simulink model "Consigna5_2_1"  (R2024b)
settings: Solver=ode45  StartTime=0.0  StopTime=20  RelTol=1e-3
values from neighbouring files (symbols this model uses):
  A_corrientes = [0 1; -omega_n_corrientes^2 -2*omega_n_corrientes]    [parametros.m]
  A_inversor = [0 1; -omega_n_inversor^2 -2*omega_n_inversor]    [parametros.m]
  A_posicion = [0 1; -omega_n_posicion^2 -2*omega_n_posicion]    [parametros.m]
  A_temp = -1/20    (= -0.05)    [parametros.m]
  alpha_cu = 3.9 *10^-3    (= 0.0039)    [parametros.m]
  B_corrientes = [0; omega_n_corrientes^2]    [parametros.m]
  b_eq = b_m + (1/r^2) * b_l    (= 2.19444444444e-05)    [parametros.m]
  B_inversor = [0; omega_n_inversor^2]    [parametros.m]
  b_l = 0.1    [parametros.m]
  b_m = 1.5 * 10^-5    (= 1.5e-05)    [parametros.m]
  B_posicion = [0; omega_n_posicion^2]    [parametros.m]
  B_temp = 1/20    (= 0.05)    [parametros.m]
  ba = J_eq*n*omega_pos    (= 0.0916527777778)    [parametros.m]
  C_corrientes = [1 0]    [parametros.m]
  C_inversor = [1 0]    [parametros.m]
  C_posicion = [1 0]    [parametros.m]
  C_temp = 1    [parametros.m]
  C_ts = 0.818    [parametros.m]
  g = 9.80665    [parametros.m]
  J_l = (m*l_cm^2 + J_cm) + (m_l * l_l^2)    (= 0.4583)    [parametros.m]
  J_m = 1.4 * 10^-5    (= 1.4e-05)    [parametros.m]
  K_e_int = 3200 ^3    (= 32768000000)    [parametros.m]
  K_e_omega = 3*3200^2    (= 30720000)    [parametros.m]
  K_e_theta = 9600    [parametros.m]
  k_l = m * l_cm + m_l* l_l    (= 1)    [parametros.m]
  Ksa = J_eq*n*(omega_pos^2)    (= 73.3222222222)    [parametros.m]
  Ksia = J_eq*(omega_pos^3)    (= 23463.1111111)    [parametros.m]
  L_d = 6.6 * 10^-3    (= 0.0066)    [parametros.m]
  L_ls = 0.8 * 10^-3    (= 0.0008)    [parametros.m]
  L_q = 5.8 * 10^-3    (= 0.0058)    [parametros.m]
  lambda_m = 0.016    [parametros.m]
  P_p = 3    [parametros.m]
  r = 120    [parametros.m]
  R_s_40 = 1.02    [parametros.m]
  R_ts_amb = 146.7    [parametros.m]
  T_sample = 1/f_sample    (= 4.53514739229e-05)    [parametros.m]
  Temp_s_ref = 20    [parametros.m]
  tm = X(1)    [parametros.m]
  tr = X(2)    [parametros.m]
  w2 = 188.49556    [parametros.m]
  x0_corrientes = [0;0]    [parametros.m]
  x0_inversor = [0;0]    [parametros.m]
  x0_posicion = [0; 0]    [parametros.m]
  x0_temp = 20    [parametros.m]
libraries: simulink x14, dspsigops x6
(part 1 of 4)
settings Model: Creator=nsorr  LastModifiedBy=nsorr
settings SolverCC: ZeroCrossAlgorithm=Adaptive
settings DebuggingCC: IgnoredZcDiagnostic=none

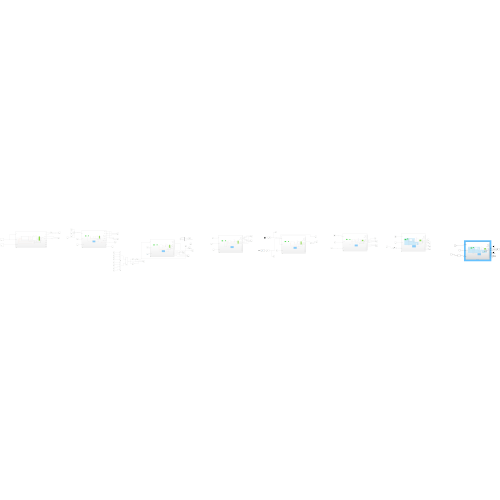
[thumbnail: Simulink's stored preview of the top-level diagram]
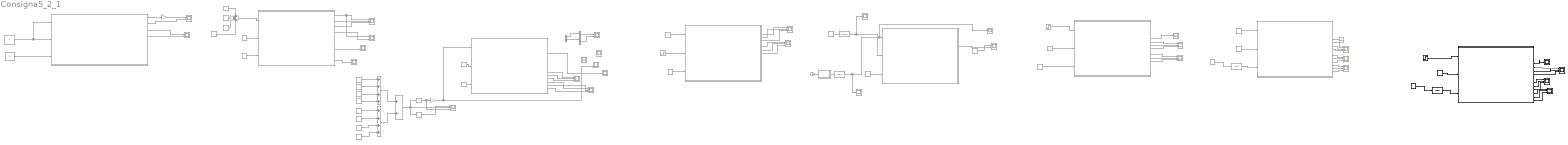
== system Consigna5_2_1 ==
  .5s : Step  Time=.5  After=5  SampleTime=0
  0-5 : simulink/Sources/Ramp  Commented=on  slope=2*pi/5  start=0  InitialOutput=0
  10-15 : simulink/Sources/Ramp  Commented=on  slope=-2*pi/5  start=10  InitialOutput=0
  5-10 : simulink/Sources/Ramp  Commented=on  slope=-2*pi/5  start=5  InitialOutput=0
  Clock : Clock  Commented=on
  Constant{,3,5..6,10,16} (6 alike) : Constant  Commented=on  Value=0
  Constant{1..2,4,7,9,11,13} (7 alike) : Constant  Commented=on  Value=20
  Constant14 : Constant  Value=20
  Constant8 : Constant  Commented=on  Value=115
  Demux2 : Demux  Commented=on  Outputs=2
  Derivative1 : Derivative  Commented=on
  Error de observador2 : Scope  Commented=on  NumInputPorts=2
  Gain : Gain  Commented=on  Gain=1/r
  Gain1 : Gain  Commented=on  Gain=1/r
  Integrator1 : Integrator  Commented=on
  MATLAB Function : MATLAB Function  Commented=on  TreatAsAtomicUnit=on
  Mux10 : Mux  Commented=on  Inputs=2
  Mux8 : Mux  Commented=on  Inputs=2
  Pulse Generator : DiscretePulseGenerator  Commented=on  PulseType=Time based  Amplitude=5  Period=1  PulseWidth=50
  Ramp : simulink/Sources/Ramp  Commented=on  slope=2*pi/5  start=15  InitialOutput=0
  Ramp1 : simulink/Sources/Ramp  Commented=on  slope=3*pi  start=5  InitialOutput=0
  Ramp10 : simulink/Sources/Ramp  Commented=on  slope=w2  start=10+tr+tm  InitialOutput=0
  Ramp11 : simulink/Sources/Ramp  Commented=on  slope=w2  start=10+tr  InitialOutput=0
  Ramp12 : simulink/Sources/Ramp  Commented=on  slope=w2  start=0  InitialOutput=0
  Ramp13 : simulink/Sources/Ramp  Commented=on  slope=-w2  start=10  InitialOutput=0
  Ramp14 : simulink/Sources/Ramp  Commented=on  slope=w2  start=5  InitialOutput=0
  Ramp15 : simulink/Sources/Ramp  Commented=on  slope=-w2  start=tr  InitialOutput=0
  Ramp16 : simulink/Sources/Ramp  Commented=on  slope=-w2  start=tr+tm  InitialOutput=0
  Ramp2 : simulink/Sources/Ramp  slope=3*pi  start=5  InitialOutput=0
  Ramp9 : simulink/Sources/Ramp  Commented=on  slope=-w2  start=15  InitialOutput=0
  Scope{,1,3..4,12} (5 alike) : Scope  Commented=on  NumInputPorts=2
  Scope{5,9..11,14,16} (6 alike) : Scope  Commented=on
  Scope{2,6..8,13,15} (6 alike) : Scope  Commented=on  NumInputPorts=3
  Scope17 : Scope  NumInputPorts=3
  Scope18 : Scope
  Step : Step  Commented=on  Time=7.5  After=5  SampleTime=0
  Step4 : Step  Commented=on  Time=7.5  After=5  SampleTime=0
  Subsystem : Subsystem  Commented=on
  Subsystem1 : Subsystem  Commented=on
  Subsystem2 : Subsystem  Commented=on
  Subsystem3 : Subsystem  Commented=on
  Subsystem4 : Subsystem  Commented=on
  Subsystem5 : Subsystem  Commented=on
  Subsystem6 : Subsystem  Commented=on
  Subsystem7 : Subsystem
  Sum : Sum  Commented=on  Inputs=++++
  Sum1 : Sum  Commented=on  Inputs=++++
  Sum2 : Sum  Commented=on  Inputs=++++
  Sum3 : Sum  Commented=on
  Transfer Fcn1 : TransferFcn  Numerator=[10]  Denominator=[1 10]
  Transfer Fcn3 : TransferFcn  Commented=on  Numerator=[100]  Denominator=[1 100]
  Transfer Fcn4 : TransferFcn  Commented=on  Numerator=[10]  Denominator=[1 10]
  Transfer Fcn8 : TransferFcn  Commented=on  Numerator=[20]  Denominator=[1 20]
  corrientes{1..4,6} (5 alike) : Scope  Commented=on  NumInputPorts=3
  corrientes5 : Scope  NumInputPorts=3
  corrientes7 : Scope  NumInputPorts=3
  posicion del brazo5 : Scope  Commented=on  NumInputPorts=2
  temp1 : Scope  Commented=on
  temp5 : Scope  Commented=on
  torque5 : Scope  Commented=on
  wires:
  Constant/1 -> Subsystem/2(T_per), Subsystem/1(Tm*)
  Constant1/1 -> Subsystem/3(T°_amb)
  Subsystem/1(T_l) -> Gain/1
  Gain/1 -> Scope/1  "T_l"
  Subsystem/2(T_m) -> Scope/2  "T_m"
  Subsystem/3(theta_m) -> Scope1/1  "theta_m"
  Subsystem/4(omega_m) -> Scope1/2  "omega_m"
  Constant2/1 -> Subsystem1/3(T°_amb)
  10-15/1 -> Sum/3
  Sum/1 -> Subsystem1/1(q1*)  "Consigna Articulación"
  Constant3/1 -> Subsystem1/2(T_per)
  0-5/1 -> Sum/1
  5-10/1 -> Sum/2
  Ramp/1 -> Sum/4
  Subsystem1/2(theta_m) -> Scope2/2  "theta_m"
  Subsystem1/7(T_m) -> Scope4/2  "Tm"
  Subsystem1/9(T_s) -> Scope5/1
  Subsystem1/4(omega_m*) -> Scope3/2  "omega_m*"
  Subsystem1/1(theta_m*) -> Scope3/1, Scope2/1  "theta_m*"
  Subsystem1/3(theta_m_obs) -> Scope2/3
  Constant4/1 -> Subsystem2/3(T°_amb)
  Constant5/1 -> Subsystem2/2(T_per)
  Ramp10/1 -> Sum1/2
  Ramp9/1 -> Sum1/1
  Ramp11/1 -> Sum1/3
  Ramp13/1 -> Sum1/4
  Ramp14/1 -> Sum2/1
  Ramp16/1 -> Sum2/2
  Ramp15/1 -> Sum2/3
  Ramp12/1 -> Sum2/4
  Sum2/1 -> Sum3/2
  Sum3/1 -> Scope8/2, Derivative1/1, Integrator1/1  "vel"
  Sum1/1 -> Sum3/1
  Integrator1/1 -> Scope8/3, Gain1/1  "Consigna de Posicion"
  Derivative1/1 -> Scope8/1  "acel"
  Mux10/1 -> Error de observador2/2
  Demux2/2 -> Mux10/1  "theta_m_obs"
  Mux8/1 -> Error de observador2/1
  Demux2/1 -> Mux8/1  "omega_m_obs"
  Subsystem2/4(T_s) -> temp5/1  "T_s"
  Gain1/1 -> posicion del brazo5/2, Subsystem2/1(q1*)
  Subsystem2/10(f_as) -> corrientes6/1  "i_as"
  Subsystem2/11(f_bs) -> corrientes6/2  "i_bs"
  Subsystem2/12(f_cs) -> corrientes6/3  "i_cs"
  Subsystem2/13(v_as) -> corrientes1/1
  Subsystem2/14(v_bs) -> corrientes1/2
  Subsystem2/15(v_cs) -> corrientes1/3
  Step4/1 -> Subsystem3/2(T_per)  "Tper"
  Constant6/1 -> Subsystem3/1(q1*)
  Constant7/1 -> Subsystem3/3(T°_amb)
  Subsystem3/8(theta_m_obs) -> Scope6/3  "theta_m_obs"
  Subsystem3/6(theta_m*) -> Scope6/1  "theta_m*"
  Subsystem3/7(theta_m) -> Scope6/2  "theta_m"
  Subsystem3/2(omega_m*) -> Scope7/1  "omega_m*"
  Subsystem3/3(omega_m) -> Scope7/2  "omega_m"
  Subsystem3/4(omega_m_obs) -> Scope7/3  "omega_m_obs"
  Clock/1 -> MATLAB Function/1(t)
  Transfer Fcn3/1 -> Scope10/1, Subsystem4/2(T_per)  "T_per"
  Constant11/1 -> Subsystem4/3(T°_amb)
  MATLAB Function/1(y) -> Transfer Fcn8/1
  Transfer Fcn8/1 -> Scope11/1, Scope9/1, Subsystem4/1(q1*)  "q1*"
  Pulse Generator/1 -> Transfer Fcn3/1  "Tper"
  Subsystem4/5(T_s) -> Scope12/2  "T_s"
  Constant8/1 -> Scope12/1  "T_Max_estator"
  Step/1 -> Subsystem5/1(T_per)  "T_per"
  Constant16/1 -> Subsystem5/3(q1*)  "q1*"
  Constant13/1 -> Subsystem5/2(T°_amb)
  Subsystem5/6(theta_m*) -> Scope13/1  "theta_m*"
  Subsystem5/7(theta_m) -> Scope13/2  "theta_m"
  Subsystem5/8(theta_m_obs) -> Scope13/3  "theta_m_obs"
  Subsystem5/10(f_as) -> corrientes2/1  "i_as"
  Subsystem5/11(f_bs) -> corrientes2/2  "i_bs"
  Subsystem5/12(f_cs) -> corrientes2/3  "i_cs"
  Subsystem5/5(T_s) -> Scope14/1  "T_s"
  Subsystem6/12(f_cs) -> corrientes3/3  "i_cs"
  Subsystem6/10(f_as) -> corrientes3/1  "i_as"
  Subsystem6/7(theta_m) -> Scope15/2  "theta_m"
  Subsystem6/8(theta_m_obs) -> Scope15/3  "theta_m_obs"
  Subsystem6/6(theta_m*) -> Scope15/1  "theta_m*"
  Subsystem6/5(T_s) -> Scope16/1  "T_s"
  Subsystem6/11(f_bs) -> corrientes3/2  "i_bs"
  Constant9/1 -> Subsystem6/2(T°_amb)
  Constant10/1 -> Subsystem6/1(T_per)
  Ramp1/1 -> Transfer Fcn4/1  "q1*"
  Transfer Fcn4/1 -> Subsystem6/3(q1*)  "q1*"
  Subsystem6/13(v_as) -> corrientes4/1  "v_as"
  Subsystem6/14(v_bs) -> corrientes4/2  "v_bs"
  Subsystem6/15(v_cs) -> corrientes4/3  "v_cs"
  Subsystem7/7(theta_m) -> Scope17/2  "theta_m"
  Subsystem7/5(T_s) -> Scope18/1  "T_s"
  Constant14/1 -> Subsystem7/2(T°_amb)
  Subsystem7/11(v_bs) -> corrientes7/2  "v_bs"
  Subsystem7/10(v_as) -> corrientes7/1  "v_as"
  Subsystem7/12(v_cs) -> corrientes7/3  "v_cs"
  Ramp2/1 -> Transfer Fcn1/1  "q1*"
  Transfer Fcn1/1 -> Subsystem7/3(q1*1)  "q1*"
  Subsystem7/6(theta_m*) -> Scope17/1  "theta_m*"
  Subsystem7/13(fas) -> corrientes5/1  "i_as"
  Subsystem7/14(fbs) -> corrientes5/2  "i_bs"
  Subsystem7/15(fcs) -> corrientes5/3  "i_cs"
  Subsystem7/8(theta_m_obs) -> Scope17/3  "theta_m_obs"
  .5s/1 -> Subsystem7/1(T_per)  "T_per"

== system Consigna5_2_1/Subsystem ==
  note: Salida medida
  note: Sensores
  note: Salida medida
  note: Salida no medida.
  Tm* : Inport
  T_per : Inport  Port=2
  T°_amb : Inport  Port=3
  Demux : Demux  Outputs=3
  Gain{,1..4} (5 alike) : Gain
  Gain5 : Gain  Gain=P_p
  Inversor: Modulador de tensión : Subsystem
  Scope : Scope
  Subsistema físico no lineal : Subsystem
      settings: PortSchema="{\"entries\":[{\"content\":{\"sides\":[{\"content\":{\"connectorIds\":[\"In1\",\"In2\",\"In3\",\"In4\",\"In5\"]},\"type\":\"ConnectorPlacement.EquallySpacedRectSide\",\"uuid\":\"67117692-d9ee-40bf-88b2-d8f6a60dc3b5\"},{\"content\":{\"connectorIds\":[\"Out1\",\"Out2\",\"Out3\"],\"side\":\"RIGHT\"},\"type\":\"ConnectorPlacement.EquallySpacedRectSide\",\"uuid\":\"ca2dbe86-e86f-47c7-8eac-1e82e6a5dbc0\"},{\"content\":{\"connectorIds\":[\"Out5\",\"Out6\",\"Out7\"],\"side\":\"TOP\"},\"type\":\"ConnectorPlacement.EquallySpacedRectSide\",\"uuid\":\"fbd4a5c3-5162-48dd-8002-932f8e6631f6\"},{\"content\":{\"connectorIds\":[\"Out4\"],\"side\":\"BOTTOM\"},\"type\":\"ConnectorPlacement.EquallySpacedRectSide\",\"uuid\":\"36392fa9-e9e5-4b1e-bf73-be72c625df16\"}]},\"type\":\"ConnectorPlacement.EquallySpacedConnector\",\"uuid\":\"e55c07f0-88b9-4508-920f-2bf50421126b\"}],\"packageUris\":[\"http://schema.mathworks.com/mf0/Connector/R2020b\"],\"version\":\"1.0\"}"
  Subsystem2 : Subsystem
  TD_PARK : MATLAB Function  TreatAsAtomicUnit=on
  TI_PARK : MATLAB Function  TreatAsAtomicUnit=on
  T_l : Outport
  T_m : Outport  Port=2
  theta_m : Outport  Port=3
  omega_m : Outport  Port=4
  T_s : Outport  Port=5
  fas : Outport  Port=6
  fbs : Outport  Port=7
  fcs : Outport  Port=8
  wires:
  Subsistema físico no lineal/3(i_abcs) -> Demux/1
  Gain5/1 -> TD_PARK/4(theta_r), TI_PARK/4(theta_r)
  T_per/1 -> Subsistema físico no lineal/1(T_per)
  Subsistema físico no lineal/6(omega_m) -> Subsystem2/2(omega_m), omega_m/1  "omega_m"
  T°_amb/1 -> Subsistema físico no lineal/5(Tº_amb)
  Gain/1 -> Scope/1, theta_m/1, Gain5/1
  Inversor: Modulador de tensión/3(v_cs) -> Subsistema físico no lineal/4(v_cs)
  Demux/3 -> Gain4/1  "i_cs"
  TI_PARK/2(fbs) -> Inversor: Modulador de tensión/2(v_bs*)
  Demux/2 -> Gain3/1  "i_bs"
  Subsistema físico no lineal/7(T_l) -> T_l/1
  Gain2/1 -> fas/1, TD_PARK/1(fas)  "i_as_medida"
  Gain4/1 -> fcs/1, TD_PARK/3(fcs)  "i_cs_medida"
  Gain1/1 -> T_s/1
  Subsistema físico no lineal/2(T_s) -> Gain1/1
  Demux/1 -> Gain2/1  "i_as"
  TI_PARK/3(fcs) -> Inversor: Modulador de tensión/3(v_cs*)
  Subsistema físico no lineal/5(T_m) -> T_m/1
  TI_PARK/1(fas) -> Inversor: Modulador de tensión/1(v_as*)
  Inversor: Modulador de tensión/1(v_as) -> Subsistema físico no lineal/2(v_as)
  Gain3/1 -> fbs/1, TD_PARK/2(fbs)  "i_bs_medida"
  Subsistema físico no lineal/1(theta_m) -> Gain/1
  Inversor: Modulador de tensión/2(v_bs) -> Subsistema físico no lineal/3(v_bs)
  Tm*/1 -> Subsystem2/1(Tm*)
  Subsistema físico no lineal/4(r_s) -> Subsystem2/3(R_s)
  TD_PARK/1(fqs) -> Subsystem2/4(i_qs^r)  "i_qs^r"
  TD_PARK/2(fds) -> Subsystem2/5(i_ds^r)  "i_ds^r"
  TD_PARK/3(f0s) -> Subsystem2/6(i_0s)  "i_0s"
  Subsystem2/1(v_qs*') -> TI_PARK/1(fqs)
  Subsystem2/2(v_ds*') -> TI_PARK/2(fds)
  Subsystem2/3(v_0s*') -> TI_PARK/3(f0s)

== system Consigna5_2_1/Subsystem1 ==
  note: Salida no medida.
  note: Salida medida
  note: Salida medida
  note: SENSORES IDEALES
  q1* : Inport
  T_per : Inport  Port=2
  T°_amb : Inport  Port=3
  Controlador PID : Subsystem
  Demux : Demux  Outputs=3
  Gain{1..5} (5 alike) : Gain
  Gain6 : Gain  Gain=P_p
  Inversor: Modulador de tensión : Subsystem
  MODULADOR DE TORQUE1 : Subsystem
  Observador de estado reducido : Subsystem
  Setpoint : Subsystem
  Subsistema físico no lineal : Subsystem
      settings: PortSchema="{\"entries\":[{\"content\":{\"sides\":[{\"content\":{\"connectorIds\":[\"In1\",\"In2\",\"In3\",\"In4\",\"In5\"]},\"type\":\"ConnectorPlacement.EquallySpacedRectSide\",\"uuid\":\"67117692-d9ee-40bf-88b2-d8f6a60dc3b5\"},{\"content\":{\"connectorIds\":[\"Out1\",\"Out2\",\"Out3\"],\"side\":\"RIGHT\"},\"type\":\"ConnectorPlacement.EquallySpacedRectSide\",\"uuid\":\"ca2dbe86-e86f-47c7-8eac-1e82e6a5dbc0\"},{\"content\":{\"connectorIds\":[\"Out4\",\"Out5\",\"Out6\"],\"side\":\"TOP\"},\"type\":\"ConnectorPlacement.EquallySpacedRectSide\",\"uuid\":\"fbd4a5c3-5162-48dd-8002-932f8e6631f6\"}]},\"type\":\"ConnectorPlacement.EquallySpacedConnector\",\"uuid\":\"e55c07f0-88b9-4508-920f-2bf50421126b\"}],\"packageUris\":[\"http://schema.mathworks.com/mf0/Connector/R2020b\"],\"version\":\"1.0\"}"
  T DE PARK DIRECTA. : MATLAB Function  TreatAsAtomicUnit=on
  T DE PARK INVERSA : MATLAB Function  TreatAsAtomicUnit=on
  theta_m* : Outport
  theta_m : Outport  Port=2
  theta_m_obs : Outport  Port=3
  omega_m* : Outport  Port=4
  omega_m : Outport  Port=5
  omega_m_obs : Outport  Port=6
  T_m : Outport  Port=7
  T_l : Outport  Port=8
  T_s : Outport  Port=9
  wires:
  Subsistema físico no lineal/6(T_l) -> T_l/1
  Demux/1 -> Gain3/1  "i_as"
  Inversor: Modulador de tensión/3(v_cs) -> Subsistema físico no lineal/4(v_cs)
  T DE PARK INVERSA/3(fcs) -> Inversor: Modulador de tensión/3(v_cs*)
  Subsistema físico no lineal/3(i_abcs) -> Demux/1
  Gain6/1 -> T DE PARK INVERSA/4(theta_r), T DE PARK DIRECTA./4(theta_r)  "theta_r"
  T DE PARK INVERSA/2(fbs) -> Inversor: Modulador de tensión/2(v_bs*)
  Gain5/1 -> T DE PARK DIRECTA./3(fcs)  "i_cs_medida"
  Inversor: Modulador de tensión/2(v_bs) -> Subsistema físico no lineal/3(v_bs)
  T°_amb/1 -> Subsistema físico no lineal/5(Tº_amb)
  MODULADOR DE TORQUE1/3(v_0s*') -> T DE PARK INVERSA/3(f0s)
  Subsistema físico no lineal/2(T_s) -> MODULADOR DE TORQUE1/6(Ts), Gain2/1
  Gain3/1 -> T DE PARK DIRECTA./1(fas)  "i_as_medida"
  T DE PARK INVERSA/1(fas) -> Inversor: Modulador de tensión/1(v_as*)
  Subsistema físico no lineal/5(T_m) -> omega_m/1
  T_per/1 -> Subsistema físico no lineal/1(T_per)
  Gain1/1 -> theta_m/1, Observador de estado reducido/2(theta_m), Gain6/1  "theta_m"
  Subsistema físico no lineal/1(theta_m) -> Gain1/1
  Gain4/1 -> T DE PARK DIRECTA./2(fbs)  "i_bs_medida"
  Subsistema físico no lineal/4(omega_m) -> T_m/1
  MODULADOR DE TORQUE1/1(v_qs*') -> T DE PARK INVERSA/1(fqs)
  Inversor: Modulador de tensión/1(v_as) -> Subsistema físico no lineal/2(v_as)
  Gain2/1 -> T_s/1
  Demux/2 -> Gain4/1  "i_bs"
  Demux/3 -> Gain5/1  "i_cs"
  MODULADOR DE TORQUE1/2(v_ds*') -> T DE PARK INVERSA/2(fds)
  ? -> ?
  Setpoint/1(theta_m*) -> theta_m*/1
  q1*/1 -> Setpoint/1(q1*)
  Controlador PID/1(Tm*) -> MODULADOR DE TORQUE1/1(Tm*)
  Setpoint/2(omega_m*) -> Controlador PID/1(omega_m*), omega_m*/1
  T DE PARK DIRECTA./2(fds) -> MODULADOR DE TORQUE1/4(i_ds^r)  "i_ds^r"
  Observador de estado reducido/1(omega_m_obs) -> omega_m_obs/1, Controlador PID/2(omega_m), MODULADOR DE TORQUE1/2(omega_m)
  T DE PARK DIRECTA./1(fqs) -> MODULADOR DE TORQUE1/3(i_qs^r)  "i_qs^r"
  T DE PARK DIRECTA./3(f0s) -> MODULADOR DE TORQUE1/5(i_0s)  "i_0s"
  Observador de estado reducido/2(theta_m_obs) -> theta_m_obs/1

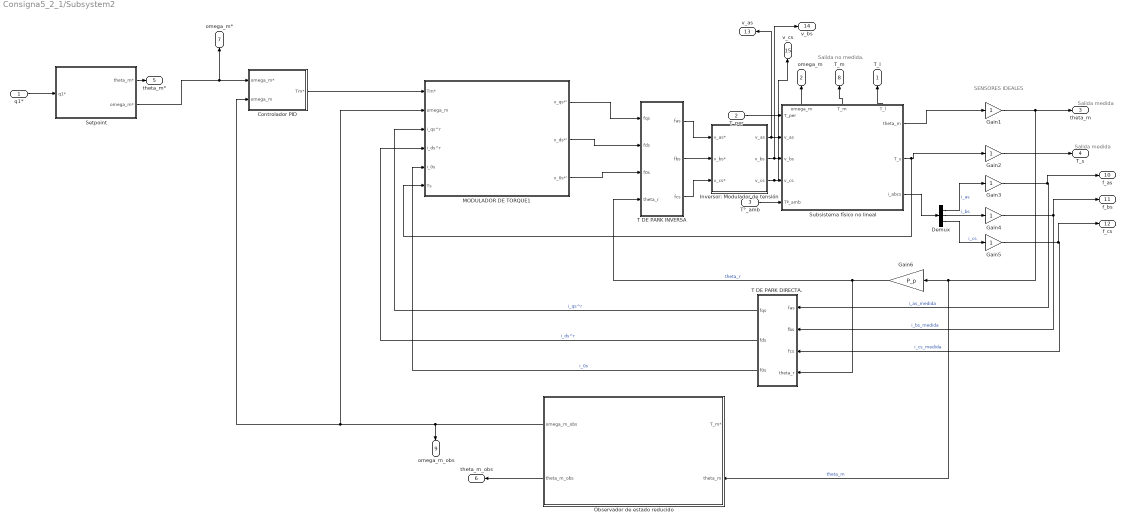
== system Consigna5_2_1/Subsystem2 ==
  note: Salida no medida.
  note: Salida medida
  note: Salida medida
  note: SENSORES IDEALES
  q1* : Inport
  T_per : Inport  Port=2
  T°_amb : Inport  Port=3
  Controlador PID : Subsystem
  Demux : Demux  Outputs=3
  Gain{1..5} (5 alike) : Gain
  Gain6 : Gain  Gain=P_p
  Inversor: Modulador de tensión : Subsystem
  MODULADOR DE TORQUE1 : Subsystem
  Observador de estado reducido : Subsystem
  Setpoint : Subsystem
  Subsistema físico no lineal : Subsystem
      settings: PortSchema="{\"entries\":[{\"content\":{\"sides\":[{\"content\":{\"connectorIds\":[\"In1\",\"In2\",\"In3\",\"In4\",\"In5\"]},\"type\":\"ConnectorPlacement.EquallySpacedRectSide\",\"uuid\":\"67117692-d9ee-40bf-88b2-d8f6a60dc3b5\"},{\"content\":{\"connectorIds\":[\"Out1\",\"Out2\",\"Out3\"],\"side\":\"RIGHT\"},\"type\":\"ConnectorPlacement.EquallySpacedRectSide\",\"uuid\":\"ca2dbe86-e86f-47c7-8eac-1e82e6a5dbc0\"},{\"content\":{\"connectorIds\":[\"Out4\",\"Out5\",\"Out6\"],\"side\":\"TOP\"},\"type\":\"ConnectorPlacement.EquallySpacedRectSide\",\"uuid\":\"fbd4a5c3-5162-48dd-8002-932f8e6631f6\"}]},\"type\":\"ConnectorPlacement.EquallySpacedConnector\",\"uuid\":\"e55c07f0-88b9-4508-920f-2bf50421126b\"}],\"packageUris\":[\"http://schema.mathworks.com/mf0/Connector/R2020b\"],\"version\":\"1.0\"}"
  T DE PARK DIRECTA. : MATLAB Function  TreatAsAtomicUnit=on
  T DE PARK INVERSA : MATLAB Function  TreatAsAtomicUnit=on
  T_l : Outport
  omega_m : Outport  Port=2
  theta_m : Outport  Port=3
  T_s : Outport  Port=4
  theta_m* : Outport  Port=5
  theta_m_obs : Outport  Port=6
  omega_m* : Outport  Port=7
  T_m : Outport  Port=8
  omega_m_obs : Outport  Port=9
  f_as : Outport  Port=10
  f_bs : Outport  Port=11
  f_cs : Outport  Port=12
  v_as : Outport  Port=13
  v_bs : Outport  Port=14
  v_cs : Outport  Port=15
  wires:
  Subsistema físico no lineal/6(T_l) -> T_l/1
  Demux/1 -> Gain3/1  "i_as"
  Inversor: Modulador de tensión/3(v_cs) -> v_cs/1, Subsistema físico no lineal/4(v_cs)
  T DE PARK INVERSA/3(fcs) -> Inversor: Modulador de tensión/3(v_cs*)
  Subsistema físico no lineal/3(i_abcs) -> Demux/1
  Gain6/1 -> T DE PARK INVERSA/4(theta_r), T DE PARK DIRECTA./4(theta_r)  "theta_r"
  T DE PARK INVERSA/2(fbs) -> Inversor: Modulador de tensión/2(v_bs*)
  Gain5/1 -> f_cs/1, T DE PARK DIRECTA./3(fcs)  "i_cs_medida"
  Inversor: Modulador de tensión/2(v_bs) -> v_bs/1, Subsistema físico no lineal/3(v_bs)
  T°_amb/1 -> Subsistema físico no lineal/5(Tº_amb)
  MODULADOR DE TORQUE1/3(v_0s*') -> T DE PARK INVERSA/3(f0s)
  Subsistema físico no lineal/2(T_s) -> MODULADOR DE TORQUE1/6(Ts), Gain2/1
  Gain3/1 -> f_as/1, T DE PARK DIRECTA./1(fas)  "i_as_medida"
  T DE PARK INVERSA/1(fas) -> Inversor: Modulador de tensión/1(v_as*)
  Subsistema físico no lineal/5(T_m) -> T_m/1
  T_per/1 -> Subsistema físico no lineal/1(T_per)
  Gain1/1 -> theta_m/1, Observador de estado reducido/2(theta_m), Gain6/1  "theta_m"
  Subsistema físico no lineal/1(theta_m) -> Gain1/1
  Gain4/1 -> f_bs/1, T DE PARK DIRECTA./2(fbs)  "i_bs_medida"
  Subsistema físico no lineal/4(omega_m) -> omega_m/1
  MODULADOR DE TORQUE1/1(v_qs*') -> T DE PARK INVERSA/1(fqs)
  Inversor: Modulador de tensión/1(v_as) -> v_as/1, Subsistema físico no lineal/2(v_as)
  Gain2/1 -> T_s/1
  Demux/2 -> Gain4/1  "i_bs"
  Demux/3 -> Gain5/1  "i_cs"
  MODULADOR DE TORQUE1/2(v_ds*') -> T DE PARK INVERSA/2(fds)
  Setpoint/1(theta_m*) -> theta_m*/1
  q1*/1 -> Setpoint/1(q1*)
  Controlador PID/1(Tm*) -> MODULADOR DE TORQUE1/1(Tm*)
  Setpoint/2(omega_m*) -> Controlador PID/1(omega_m*), omega_m*/1
  T DE PARK DIRECTA./2(fds) -> MODULADOR DE TORQUE1/4(i_ds^r)  "i_ds^r"
  Observador de estado reducido/1(omega_m_obs) -> omega_m_obs/1, Controlador PID/2(omega_m), MODULADOR DE TORQUE1/2(omega_m)
  T DE PARK DIRECTA./1(fqs) -> MODULADOR DE TORQUE1/3(i_qs^r)  "i_qs^r"
  T DE PARK DIRECTA./3(f0s) -> MODULADOR DE TORQUE1/5(i_0s)  "i_0s"
  Observador de estado reducido/2(theta_m_obs) -> theta_m_obs/1

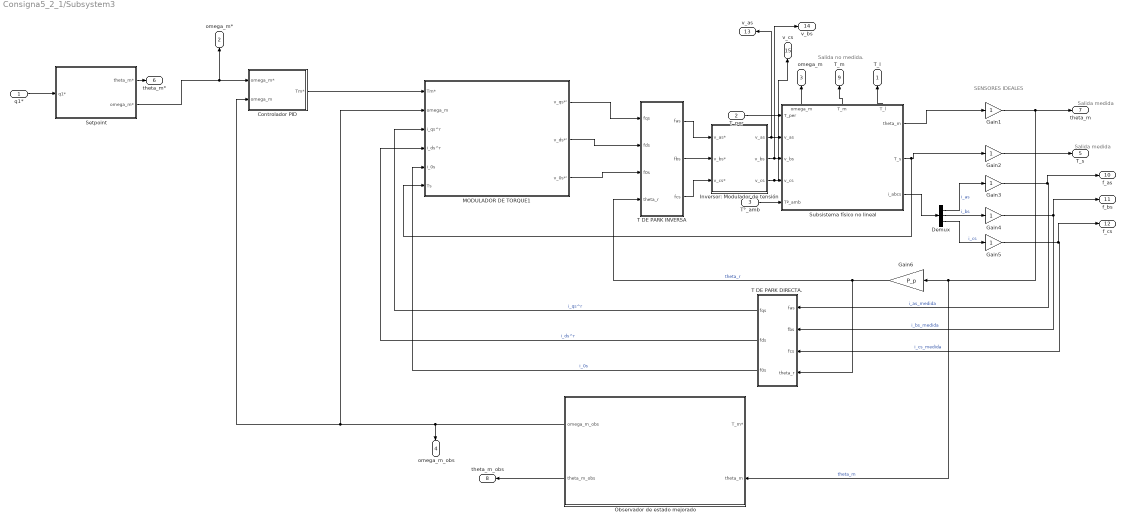
== system Consigna5_2_1/Subsystem3 ==
  note: Salida no medida.
  note: Salida medida
  note: Salida medida
  note: SENSORES IDEALES
  q1* : Inport
  T_per : Inport  Port=2
  T°_amb : Inport  Port=3
  Controlador PID : Subsystem
  Demux : Demux  Outputs=3
  Gain{1..5} (5 alike) : Gain
  Gain6 : Gain  Gain=P_p
  Inversor: Modulador de tensión : Subsystem
  MODULADOR DE TORQUE1 : Subsystem
  Observador de estado mejorado : Subsystem
  Setpoint : Subsystem
  Subsistema físico no lineal : Subsystem
      settings: PortSchema="{\"entries\":[{\"content\":{\"sides\":[{\"content\":{\"connectorIds\":[\"In1\",\"In2\",\"In3\",\"In4\",\"In5\"]},\"type\":\"ConnectorPlacement.EquallySpacedRectSide\",\"uuid\":\"67117692-d9ee-40bf-88b2-d8f6a60dc3b5\"},{\"content\":{\"connectorIds\":[\"Out1\",\"Out2\",\"Out3\"],\"side\":\"RIGHT\"},\"type\":\"ConnectorPlacement.EquallySpacedRectSide\",\"uuid\":\"ca2dbe86-e86f-47c7-8eac-1e82e6a5dbc0\"},{\"content\":{\"connectorIds\":[\"Out4\",\"Out5\",\"Out6\"],\"side\":\"TOP\"},\"type\":\"ConnectorPlacement.EquallySpacedRectSide\",\"uuid\":\"fbd4a5c3-5162-48dd-8002-932f8e6631f6\"}]},\"type\":\"ConnectorPlacement.EquallySpacedConnector\",\"uuid\":\"e55c07f0-88b9-4508-920f-2bf50421126b\"}],\"packageUris\":[\"http://schema.mathworks.com/mf0/Connector/R2020b\"],\"version\":\"1.0\"}"
  T DE PARK DIRECTA. : MATLAB Function  TreatAsAtomicUnit=on
  T DE PARK INVERSA : MATLAB Function  TreatAsAtomicUnit=on
  T_l : Outport
  omega_m* : Outport  Port=2
  omega_m : Outport  Port=3
  omega_m_obs : Outport  Port=4
  T_s : Outport  Port=5
  theta_m* : Outport  Port=6
  theta_m : Outport  Port=7
  theta_m_obs : Outport  Port=8
  T_m : Outport  Port=9
  f_as : Outport  Port=10
  f_bs : Outport  Port=11
  f_cs : Outport  Port=12
  v_as : Outport  Port=13
  v_bs : Outport  Port=14
  v_cs : Outport  Port=15
  wires:
  Subsistema físico no lineal/6(T_l) -> T_l/1
  Demux/1 -> Gain3/1  "i_as"
  Inversor: Modulador de tensión/3(v_cs) -> v_cs/1, Subsistema físico no lineal/4(v_cs)
  T DE PARK INVERSA/3(fcs) -> Inversor: Modulador de tensión/3(v_cs*)
  Subsistema físico no lineal/3(i_abcs) -> Demux/1
  Gain6/1 -> T DE PARK INVERSA/4(theta_r), T DE PARK DIRECTA./4(theta_r)  "theta_r"
  T DE PARK INVERSA/2(fbs) -> Inversor: Modulador de tensión/2(v_bs*)
  Gain5/1 -> f_cs/1, T DE PARK DIRECTA./3(fcs)  "i_cs_medida"
  Inversor: Modulador de tensión/2(v_bs) -> v_bs/1, Subsistema físico no lineal/3(v_bs)
  T°_amb/1 -> Subsistema físico no lineal/5(Tº_amb)
  MODULADOR DE TORQUE1/3(v_0s*') -> T DE PARK INVERSA/3(f0s)
  Subsistema físico no lineal/2(T_s) -> MODULADOR DE TORQUE1/6(Ts), Gain2/1
  Gain3/1 -> f_as/1, T DE PARK DIRECTA./1(fas)  "i_as_medida"
  T DE PARK INVERSA/1(fas) -> Inversor: Modulador de tensión/1(v_as*)
  Subsistema físico no lineal/5(T_m) -> T_m/1
  T_per/1 -> Subsistema físico no lineal/1(T_per)
  Gain1/1 -> theta_m/1, Observador de estado mejorado/2(theta_m), Gain6/1  "theta_m"
  Subsistema físico no lineal/1(theta_m) -> Gain1/1
  Gain4/1 -> f_bs/1, T DE PARK DIRECTA./2(fbs)  "i_bs_medida"
  Subsistema físico no lineal/4(omega_m) -> omega_m/1
  MODULADOR DE TORQUE1/1(v_qs*') -> T DE PARK INVERSA/1(fqs)
  Inversor: Modulador de tensión/1(v_as) -> v_as/1, Subsistema físico no lineal/2(v_as)
  Gain2/1 -> T_s/1
  Demux/2 -> Gain4/1  "i_bs"
  Demux/3 -> Gain5/1  "i_cs"
  MODULADOR DE TORQUE1/2(v_ds*') -> T DE PARK INVERSA/2(fds)
  Setpoint/1(theta_m*) -> theta_m*/1
  q1*/1 -> Setpoint/1(q1*)
  Controlador PID/1(Tm*) -> MODULADOR DE TORQUE1/1(Tm*)
  Setpoint/2(omega_m*) -> Controlador PID/1(omega_m*), omega_m*/1
  T DE PARK DIRECTA./2(fds) -> MODULADOR DE TORQUE1/4(i_ds^r)  "i_ds^r"
  Observador de estado mejorado/1(omega_m_obs) -> omega_m_obs/1, Controlador PID/2(omega_m), MODULADOR DE TORQUE1/2(omega_m)
  T DE PARK DIRECTA./1(fqs) -> MODULADOR DE TORQUE1/3(i_qs^r)  "i_qs^r"
  T DE PARK DIRECTA./3(f0s) -> MODULADOR DE TORQUE1/5(i_0s)  "i_0s"
  Observador de estado mejorado/2(theta_m_obs) -> theta_m_obs/1

== system Consigna5_2_1/Subsystem4 ==
  note: Salida no medida.
  note: Salida medida
  note: Salida medida
  note: SENSORES IDEALES
  q1* : Inport
  T_per : Inport  Port=2
  T°_amb : Inport  Port=3
  Controlador PID : Subsystem
  Demux : Demux  Outputs=3
  Gain{1..5} (5 alike) : Gain
  Gain6 : Gain  Gain=P_p
  Inversor: Modulador de tensión : Subsystem
  MODULADOR DE TORQUE1 : Subsystem
  Observador de estado mejorado : Subsystem
  Setpoint : Subsystem
  Subsistema físico no lineal : Subsystem
      settings: PortSchema="{\"entries\":[{\"content\":{\"sides\":[{\"content\":{\"connectorIds\":[\"In1\",\"In2\",\"In3\",\"In4\",\"In5\"]},\"type\":\"ConnectorPlacement.EquallySpacedRectSide\",\"uuid\":\"67117692-d9ee-40bf-88b2-d8f6a60dc3b5\"},{\"content\":{\"connectorIds\":[\"Out1\",\"Out2\",\"Out3\"],\"side\":\"RIGHT\"},\"type\":\"ConnectorPlacement.EquallySpacedRectSide\",\"uuid\":\"ca2dbe86-e86f-47c7-8eac-1e82e6a5dbc0\"},{\"content\":{\"connectorIds\":[\"Out4\",\"Out5\",\"Out6\"],\"side\":\"TOP\"},\"type\":\"ConnectorPlacement.EquallySpacedRectSide\",\"uuid\":\"fbd4a5c3-5162-48dd-8002-932f8e6631f6\"}]},\"type\":\"ConnectorPlacement.EquallySpacedConnector\",\"uuid\":\"e55c07f0-88b9-4508-920f-2bf50421126b\"}],\"packageUris\":[\"http://schema.mathworks.com/mf0/Connector/R2020b\"],\"version\":\"1.0\"}"
  T DE PARK DIRECTA. : MATLAB Function  TreatAsAtomicUnit=on
  T DE PARK INVERSA : MATLAB Function  TreatAsAtomicUnit=on
  T_l : Outport
  omega_m* : Outport  Port=2
  omega_m : Outport  Port=3
  omega_m_obs : Outport  Port=4
  T_s : Outport  Port=5
  theta_m* : Outport  Port=6
  theta_m : Outport  Port=7
  theta_m_obs : Outport  Port=8
  T_m : Outport  Port=9
  f_as : Outport  Port=10
  f_bs : Outport  Port=11
  f_cs : Outport  Port=12
  v_as : Outport  Port=13
  v_bs : Outport  Port=14
  v_cs : Outport  Port=15
  wires:
  Subsistema físico no lineal/6(T_l) -> T_l/1
  Demux/1 -> Gain3/1  "i_as"
  Inversor: Modulador de tensión/3(v_cs) -> v_cs/1, Subsistema físico no lineal/4(v_cs)
  T DE PARK INVERSA/3(fcs) -> Inversor: Modulador de tensión/3(v_cs*)
  Subsistema físico no lineal/3(i_abcs) -> Demux/1
  Gain6/1 -> T DE PARK INVERSA/4(theta_r), T DE PARK DIRECTA./4(theta_r)  "theta_r"
  T DE PARK INVERSA/2(fbs) -> Inversor: Modulador de tensión/2(v_bs*)
  Gain5/1 -> f_cs/1, T DE PARK DIRECTA./3(fcs)  "i_cs_medida"
  Inversor: Modulador de tensión/2(v_bs) -> v_bs/1, Subsistema físico no lineal/3(v_bs)
  T°_amb/1 -> Subsistema físico no lineal/5(Tº_amb)
  MODULADOR DE TORQUE1/3(v_0s*') -> T DE PARK INVERSA/3(f0s)
  Subsistema físico no lineal/2(T_s) -> MODULADOR DE TORQUE1/6(Ts), Gain2/1
  Gain3/1 -> f_as/1, T DE PARK DIRECTA./1(fas)  "i_as_medida"
  T DE PARK INVERSA/1(fas) -> Inversor: Modulador de tensión/1(v_as*)
  Subsistema físico no lineal/5(T_m) -> T_m/1
  T_per/1 -> Subsistema físico no lineal/1(T_per)
  Gain1/1 -> theta_m/1, Observador de estado mejorado/2(theta_m), Gain6/1  "theta_m"
  Subsistema físico no lineal/1(theta_m) -> Gain1/1
  Gain4/1 -> f_bs/1, T DE PARK DIRECTA./2(fbs)  "i_bs_medida"
  Subsistema físico no lineal/4(omega_m) -> omega_m/1
  MODULADOR DE TORQUE1/1(v_qs*') -> T DE PARK INVERSA/1(fqs)
  Inversor: Modulador de tensión/1(v_as) -> v_as/1, Subsistema físico no lineal/2(v_as)
  Gain2/1 -> T_s/1
  Demux/2 -> Gain4/1  "i_bs"
  Demux/3 -> Gain5/1  "i_cs"
  MODULADOR DE TORQUE1/2(v_ds*') -> T DE PARK INVERSA/2(fds)
  Setpoint/1(theta_m*) -> theta_m*/1
  q1*/1 -> Setpoint/1(q1*)
  Controlador PID/1(Tm*) -> MODULADOR DE TORQUE1/1(Tm*)
  Setpoint/2(omega_m*) -> Controlador PID/1(omega_m*), omega_m*/1
  T DE PARK DIRECTA./2(fds) -> MODULADOR DE TORQUE1/4(i_ds^r)  "i_ds^r"
  Observador de estado mejorado/1(omega_m_obs) -> omega_m_obs/1, Controlador PID/2(omega_m), MODULADOR DE TORQUE1/2(omega_m)
  T DE PARK DIRECTA./1(fqs) -> MODULADOR DE TORQUE1/3(i_qs^r)  "i_qs^r"
  T DE PARK DIRECTA./3(f0s) -> MODULADOR DE TORQUE1/5(i_0s)  "i_0s"
  Observador de estado mejorado/2(theta_m_obs) -> theta_m_obs/1

== system Consigna5_2_1/Subsystem5 ==
  note: Salida no medida.
  note: Salida medida
  note: Salida medida
  T_per : Inport
  T°_amb : Inport  Port=2
  q1* : Inport  Port=3
  Controlador PID : Subsystem
  Demux : Demux  Outputs=3
  Gain6 : Gain  Gain=P_p
  Inversor: Modulador de tensión : Subsystem
  MODULADOR DE TORQUE1 : Subsystem
  Observador de estado mejorado : Subsystem
  Sensores : Subsystem
  Setpoint : Subsystem
  Subsistema físico no lineal : Subsystem
      settings: PortSchema="{\"entries\":[{\"content\":{\"sides\":[{\"content\":{\"connectorIds\":[\"In1\",\"In2\",\"In3\",\"In4\",\"In5\"]},\"type\":\"ConnectorPlacement.EquallySpacedRectSide\",\"uuid\":\"67117692-d9ee-40bf-88b2-d8f6a60dc3b5\"},{\"content\":{\"connectorIds\":[\"Out1\",\"Out2\",\"Out3\"],\"side\":\"RIGHT\"},\"type\":\"ConnectorPlacement.EquallySpacedRectSide\",\"uuid\":\"ca2dbe86-e86f-47c7-8eac-1e82e6a5dbc0\"},{\"content\":{\"connectorIds\":[\"Out4\",\"Out5\",\"Out6\"],\"side\":\"TOP\"},\"type\":\"ConnectorPlacement.EquallySpacedRectSide\",\"uuid\":\"fbd4a5c3-5162-48dd-8002-932f8e6631f6\"}]},\"type\":\"ConnectorPlacement.EquallySpacedConnector\",\"uuid\":\"e55c07f0-88b9-4508-920f-2bf50421126b\"}],\"packageUris\":[\"http://schema.mathworks.com/mf0/Connector/R2020b\"],\"version\":\"1.0\"}"
  T DE PARK DIRECTA. : MATLAB Function  TreatAsAtomicUnit=on
  T DE PARK INVERSA : MATLAB Function  TreatAsAtomicUnit=on
  T_l : Outport
  omega_m* : Outport  Port=2
  omega_m : Outport  Port=3
  omega_m_obs : Outport  Port=4
  T_s : Outport  Port=5
  theta_m* : Outport  Port=6
  theta_m : Outport  Port=7
  theta_m_obs : Outport  Port=8
  T_m : Outport  Port=9
  f_as : Outport  Port=10
  f_bs : Outport  Port=11
  f_cs : Outport  Port=12
  v_as : Outport  Port=13
  v_bs : Outport  Port=14
  v_cs : Outport  Port=15
  wires:
  Subsistema físico no lineal/6(T_l) -> T_l/1
  Demux/1 -> Sensores/3(i_as)  "i_as"
  Inversor: Modulador de tensión/3(v_cs) -> v_cs/1, Subsistema físico no lineal/4(v_cs)
  T DE PARK INVERSA/3(fcs) -> Inversor: Modulador de tensión/3(v_cs*)
  Subsistema físico no lineal/3(i_abcs) -> Demux/1
  Gain6/1 -> T DE PARK INVERSA/4(theta_r), T DE PARK DIRECTA./4(theta_r)  "theta_r"
  T DE PARK INVERSA/2(fbs) -> Inversor: Modulador de tensión/2(v_bs*)
  Sensores/5(i_cs_medida) -> T DE PARK DIRECTA./3(fcs), f_cs/1  "i_cs_medida"
  Inversor: Modulador de tensión/2(v_bs) -> v_bs/1, Subsistema físico no lineal/3(v_bs)
  T°_amb/1 -> Subsistema físico no lineal/5(Tº_amb)
  MODULADOR DE TORQUE1/3(v_0s*') -> T DE PARK INVERSA/3(f0s)
  Subsistema físico no lineal/2(T_s) -> Sensores/2(T_s), MODULADOR DE TORQUE1/6(Ts)
  Sensores/3(i_as_medida) -> T DE PARK DIRECTA./1(fas), f_as/1  "i_as_medida"
  T DE PARK INVERSA/1(fas) -> Inversor: Modulador de tensión/1(v_as*)
  Subsistema físico no lineal/5(T_m) -> T_m/1
  T_per/1 -> Subsistema físico no lineal/1(T_per)
  Sensores/1(theta_m_medida) -> Observador de estado mejorado/2(theta_m), Gain6/1, theta_m/1  "theta_m"
  Subsistema físico no lineal/1(theta_m) -> Sensores/1(theta_m)
  Sensores/4(i_bs_medida) -> T DE PARK DIRECTA./2(fbs), f_bs/1  "i_bs_medida"
  Subsistema físico no lineal/4(omega_m) -> omega_m/1
  MODULADOR DE TORQUE1/1(v_qs*') -> T DE PARK INVERSA/1(fqs)
  Inversor: Modulador de tensión/1(v_as) -> v_as/1, Subsistema físico no lineal/2(v_as)
  Sensores/2(T_s_medida) -> T_s/1
  Demux/2 -> Sensores/4(i_bs)  "i_bs"
  Demux/3 -> Sensores/5(i_cs)  "i_cs"
  MODULADOR DE TORQUE1/2(v_ds*') -> T DE PARK INVERSA/2(fds)
  Setpoint/1(theta_m*) -> theta_m*/1
  q1*/1 -> Setpoint/1(q1*)
  Controlador PID/1(Tm*) -> MODULADOR DE TORQUE1/1(Tm*)
  Setpoint/2(omega_m*) -> Controlador PID/1(omega_m*), omega_m*/1
  T DE PARK DIRECTA./2(fds) -> MODULADOR DE TORQUE1/4(i_ds^r)  "i_ds^r"
  Observador de estado mejorado/1(omega_m_obs) -> omega_m_obs/1, Controlador PID/2(omega_m), MODULADOR DE TORQUE1/2(omega_m)
  T DE PARK DIRECTA./1(fqs) -> MODULADOR DE TORQUE1/3(i_qs^r)  "i_qs^r"
  T DE PARK DIRECTA./3(f0s) -> MODULADOR DE TORQUE1/5(i_0s)  "i_0s"
  Observador de estado mejorado/2(theta_m_obs) -> theta_m_obs/1

== system Consigna5_2_1/Subsystem6 ==
  note: Salida no medida.
  note: Salida medida
  note: Salida medida
  note: CONTROLADOR
  T_per : Inport
  T°_amb : Inport  Port=2
  q1* : Inport  Port=3
  CONTROLADOR PID : Subsystem
  Demux : Demux  Outputs=3
  Gain6 : Gain  Gain=P_p
  MODULADOR DE TORQUE1 : Subsystem
  MODULAR DE TENSIÓN NO IDEAL : Subsystem
  OBSERVADOR DE ESTADO MEJORADO : Subsystem
  PLANTA : Subsystem
      settings: PortSchema="{\"entries\":[{\"content\":{\"sides\":[{\"content\":{\"connectorIds\":[\"In1\",\"In2\",\"In3\",\"In4\",\"In5\"]},\"type\":\"ConnectorPlacement.EquallySpacedRectSide\",\"uuid\":\"67117692-d9ee-40bf-88b2-d8f6a60dc3b5\"},{\"content\":{\"connectorIds\":[\"Out1\",\"Out2\",\"Out3\"],\"side\":\"RIGHT\"},\"type\":\"ConnectorPlacement.EquallySpacedRectSide\",\"uuid\":\"ca2dbe86-e86f-47c7-8eac-1e82e6a5dbc0\"},{\"content\":{\"connectorIds\":[\"Out4\",\"Out5\",\"Out6\"],\"side\":\"TOP\"},\"type\":\"ConnectorPlacement.EquallySpacedRectSide\",\"uuid\":\"fbd4a5c3-5162-48dd-8002-932f8e6631f6\"}]},\"type\":\"ConnectorPlacement.EquallySpacedConnector\",\"uuid\":\"e55c07f0-88b9-4508-920f-2bf50421126b\"}],\"packageUris\":[\"http://schema.mathworks.com/mf0/Connector/R2020b\"],\"version\":\"1.0\"}"
  SENSORES NO IDEALES : Subsystem
  SETPOINT : Subsystem
  T DE PARK DIRECTA. : MATLAB Function  TreatAsAtomicUnit=on
  T DE PARK INVERSA : MATLAB Function  TreatAsAtomicUnit=on
  T_l : Outport
  omega_m* : Outport  Port=2
  omega_m : Outport  Port=3
  omega_m_obs : Outport  Port=4
  T_s : Outport  Port=5
  theta_m* : Outport  Port=6
  theta_m : Outport  Port=7
  theta_m_obs : Outport  Port=8
  T_m : Outport  Port=9
  f_as : Outport  Port=10
  f_bs : Outport  Port=11
  f_cs : Outport  Port=12
  v_as : Outport  Port=13
  v_bs : Outport  Port=14
  v_cs : Outport  Port=15
  wires:
  PLANTA/6(T_l) -> T_l/1
  Demux/1 -> SENSORES NO IDEALES/3(i_as)  "i_as"
  MODULAR DE TENSIÓN NO IDEAL/3(v_cs) -> v_cs/1, PLANTA/4(v_cs)
  T DE PARK INVERSA/3(fcs) -> MODULAR DE TENSIÓN NO IDEAL/3(v_cs*)
  PLANTA/3(i_abcs) -> Demux/1
  Gain6/1 -> T DE PARK INVERSA/4(theta_r), T DE PARK DIRECTA./4(theta_r)  "theta_r"
  T DE PARK INVERSA/2(fbs) -> MODULAR DE TENSIÓN NO IDEAL/2(v_bs*)
  SENSORES NO IDEALES/5(i_cs_medida) -> T DE PARK DIRECTA./3(fcs), f_cs/1  "i_cs_medida"
  MODULAR DE TENSIÓN NO IDEAL/2(v_bs) -> v_bs/1, PLANTA/3(v_bs)
  T°_amb/1 -> PLANTA/5(Tº_amb)
  MODULADOR DE TORQUE1/3(v_0s*') -> T DE PARK INVERSA/3(f0s)
  PLANTA/2(T_s) -> SENSORES NO IDEALES/2(T_s), MODULADOR DE TORQUE1/6(Ts)
  SENSORES NO IDEALES/3(i_as_medida) -> T DE PARK DIRECTA./1(fas), f_as/1  "i_as_medida"
  T DE PARK INVERSA/1(fas) -> MODULAR DE TENSIÓN NO IDEAL/1(v_as*)
  PLANTA/5(T_m) -> T_m/1
  T_per/1 -> PLANTA/1(T_per)
  SENSORES NO IDEALES/1(theta_m_medida) -> OBSERVADOR DE ESTADO MEJORADO/2(theta_m), Gain6/1, theta_m/1  "theta_m"
  PLANTA/1(theta_m) -> SENSORES NO IDEALES/1(theta_m)
  SENSORES NO IDEALES/4(i_bs_medida) -> T DE PARK DIRECTA./2(fbs), f_bs/1  "i_bs_medida"
  PLANTA/4(omega_m) -> omega_m/1
  MODULADOR DE TORQUE1/1(v_qs*') -> T DE PARK INVERSA/1(fqs)
  MODULAR DE TENSIÓN NO IDEAL/1(v_as) -> v_as/1, PLANTA/2(v_as)
  SENSORES NO IDEALES/2(T_s_medida) -> T_s/1
  Demux/2 -> SENSORES NO IDEALES/4(i_bs)  "i_bs"
  Demux/3 -> SENSORES NO IDEALES/5(i_cs)  "i_cs"
  MODULADOR DE TORQUE1/2(v_ds*') -> T DE PARK INVERSA/2(fds)
  SETPOINT/1(theta_m*) -> theta_m*/1
  q1*/1 -> SETPOINT/1(q1*)
  CONTROLADOR PID/1(Tm*) -> MODULADOR DE TORQUE1/1(Tm*)
  SETPOINT/2(omega_m*) -> omega_m*/1, CONTROLADOR PID/1(omega_m*)
  T DE PARK DIRECTA./2(fds) -> MODULADOR DE TORQUE1/4(i_ds^r)  "i_ds^r"
  OBSERVADOR DE ESTADO MEJORADO/1(omega_m_obs) -> CONTROLADOR PID/2(omega_m), MODULADOR DE TORQUE1/2(omega_m), omega_m_obs/1
  T DE PARK DIRECTA./1(fqs) -> MODULADOR DE TORQUE1/3(i_qs^r)  "i_qs^r"
  T DE PARK DIRECTA./3(f0s) -> MODULADOR DE TORQUE1/5(i_0s)  "i_0s"
  OBSERVADOR DE ESTADO MEJORADO/2(theta_m_obs) -> theta_m_obs/1

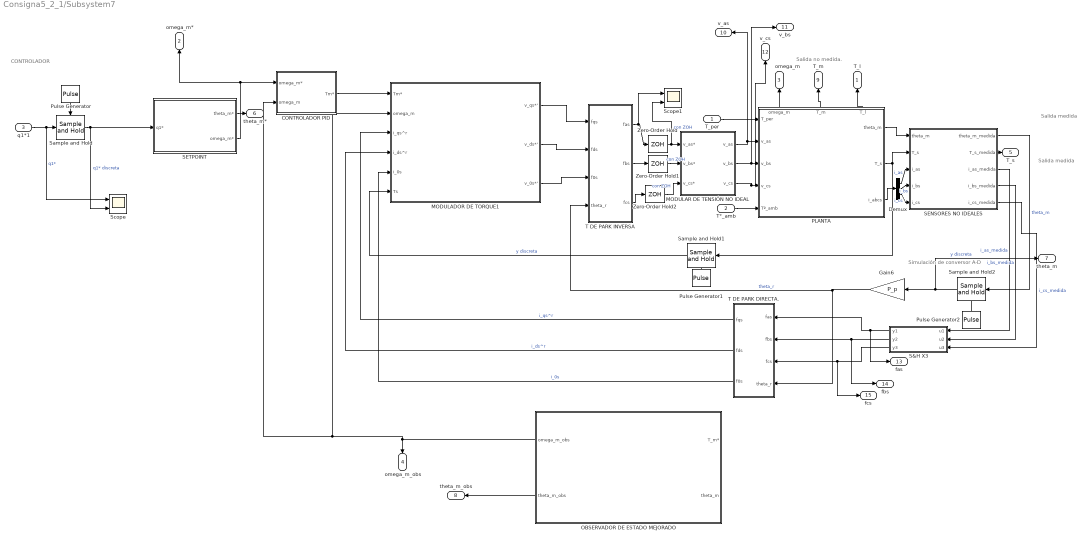
== system Consigna5_2_1/Subsystem7 ==
  note: Salida no medida.
  note: Salida medida
  note: Salida medida
  note: CONTROLADOR
  note: Simulación de conversor A-D
  T_per : Inport
  T°_amb : Inport  Port=2
  q1*1 : Inport  Port=3
  CONTROLADOR PID : Subsystem
  Demux : Demux  Outputs=3
  Gain6 : Gain  Gain=P_p
  MODULADOR DE TORQUE1 : Subsystem
  MODULAR DE TENSIÓN NO IDEAL : Subsystem
  OBSERVADOR DE ESTADO MEJORADO : Subsystem
  PLANTA : Subsystem
      settings: PortSchema="{\"entries\":[{\"content\":{\"sides\":[{\"content\":{\"connectorIds\":[\"In1\",\"In2\",\"In3\",\"In4\",\"In5\"]},\"type\":\"ConnectorPlacement.EquallySpacedRectSide\",\"uuid\":\"67117692-d9ee-40bf-88b2-d8f6a60dc3b5\"},{\"content\":{\"connectorIds\":[\"Out1\",\"Out2\",\"Out3\"],\"side\":\"RIGHT\"},\"type\":\"ConnectorPlacement.EquallySpacedRectSide\",\"uuid\":\"ca2dbe86-e86f-47c7-8eac-1e82e6a5dbc0\"},{\"content\":{\"connectorIds\":[\"Out4\",\"Out5\",\"Out6\"],\"side\":\"TOP\"},\"type\":\"ConnectorPlacement.EquallySpacedRectSide\",\"uuid\":\"fbd4a5c3-5162-48dd-8002-932f8e6631f6\"}]},\"type\":\"ConnectorPlacement.EquallySpacedConnector\",\"uuid\":\"e55c07f0-88b9-4508-920f-2bf50421126b\"}],\"packageUris\":[\"http://schema.mathworks.com/mf0/Connector/R2020b\"],\"version\":\"1.0\"}"
  Pulse Generator : DiscretePulseGenerator  PulseType=Time based  Period=T_sample  PulseWidth=50
  Pulse Generator1 : DiscretePulseGenerator  PulseType=Time based  Period=T_sample  PulseWidth=50
  Pulse Generator2 : DiscretePulseGenerator  PulseType=Time based  Period=T_sample  PulseWidth=50
  S&H X3 : Subsystem
  SENSORES NO IDEALES : Subsystem
  SETPOINT : Subsystem
  Sample and Hold : dspsigops/Sample and Hold  trig=Rising edge  initCond=0  latchinput=off
  Sample and Hold1 : dspsigops/Sample and Hold  trig=Rising edge  initCond=0  latchinput=off
  Sample and Hold2 : dspsigops/Sample and Hold  trig=Rising edge  initCond=0  latchinput=off
  Scope : Scope  NumInputPorts=2
  Scope1 : Scope  NumInputPorts=2
  T DE PARK DIRECTA. : MATLAB Function  TreatAsAtomicUnit=on
  T DE PARK INVERSA : MATLAB Function  TreatAsAtomicUnit=on
  Zero-Order Hold : ZeroOrderHold  SampleTime=T_sample
  Zero-Order Hold1 : ZeroOrderHold  SampleTime=T_sample
  Zero-Order Hold2 : ZeroOrderHold  SampleTime=T_sample
  T_l : Outport
  omega_m* : Outport  Port=2
  omega_m : Outport  Port=3
  omega_m_obs : Outport  Port=4
  T_s : Outport  Port=5
  theta_m* : Outport  Port=6
  theta_m : Outport  Port=7
  theta_m_obs : Outport  Port=8
  T_m : Outport  Port=9
  v_as : Outport  Port=10
  v_bs : Outport  Port=11
  v_cs : Outport  Port=12
  fas : Outport  Port=13
  fbs : Outport  Port=14
  fcs : Outport  Port=15
  wires:
  PLANTA/6(T_l) -> T_l/1
  Demux/1 -> SENSORES NO IDEALES/3(i_as)  "i_as"
  MODULAR DE TENSIÓN NO IDEAL/3(v_cs) -> v_cs/1, PLANTA/4(v_cs)
  PLANTA/3(i_abcs) -> Demux/1
  Gain6/1 -> T DE PARK INVERSA/4(theta_r), T DE PARK DIRECTA./4(theta_r)  "theta_r"
  SENSORES NO IDEALES/5(i_cs_medida) -> S&H X3/3(u3)  "i_cs_medida"
  MODULAR DE TENSIÓN NO IDEAL/2(v_bs) -> v_bs/1, PLANTA/3(v_bs)
  T°_amb/1 -> PLANTA/5(Tº_amb)
  MODULADOR DE TORQUE1/3(v_0s*') -> T DE PARK INVERSA/3(f0s)
  PLANTA/2(T_s) -> Sample and Hold1/1, SENSORES NO IDEALES/2(T_s)
  SENSORES NO IDEALES/3(i_as_medida) -> S&H X3/1(u1)  "i_as_medida"
  PLANTA/5(T_m) -> T_m/1
  T_per/1 -> PLANTA/1(T_per)
  SENSORES NO IDEALES/1(theta_m_medida) -> Sample and Hold2/1  "theta_m"
  PLANTA/1(theta_m) -> SENSORES NO IDEALES/1(theta_m)
  SENSORES NO IDEALES/4(i_bs_medida) -> S&H X3/2(u2)  "i_bs_medida"
  PLANTA/4(omega_m) -> omega_m/1
  MODULADOR DE TORQUE1/1(v_qs*') -> T DE PARK INVERSA/1(fqs)
  MODULAR DE TENSIÓN NO IDEAL/1(v_as) -> v_as/1, PLANTA/2(v_as)
  SENSORES NO IDEALES/2(T_s_medida) -> T_s/1
  Demux/2 -> SENSORES NO IDEALES/4(i_bs)  "i_bs"
  Demux/3 -> SENSORES NO IDEALES/5(i_cs)  "i_cs"
  MODULADOR DE TORQUE1/2(v_ds*') -> T DE PARK INVERSA/2(fds)
  SETPOINT/1(theta_m*) -> theta_m*/1
  CONTROLADOR PID/1(Tm*) -> MODULADOR DE TORQUE1/1(Tm*)
  SETPOINT/2(omega_m*) -> omega_m*/1, CONTROLADOR PID/1(omega_m*)
  T DE PARK DIRECTA./2(fds) -> MODULADOR DE TORQUE1/4(i_ds^r)  "i_ds^r"
  OBSERVADOR DE ESTADO MEJORADO/1(omega_m_obs) -> CONTROLADOR PID/2(omega_m), MODULADOR DE TORQUE1/2(omega_m), omega_m_obs/1
  T DE PARK DIRECTA./1(fqs) -> MODULADOR DE TORQUE1/3(i_qs^r)  "i_qs^r"
  T DE PARK DIRECTA./3(f0s) -> MODULADOR DE TORQUE1/5(i_0s)  "i_0s"
  OBSERVADOR DE ESTADO MEJORADO/2(theta_m_obs) -> theta_m_obs/1
  Pulse Generator/1 -> Sample and Hold/Trigger
  Sample and Hold/1 -> SETPOINT/1(q1*), Scope/2  "q1* discreta"
  q1*1/1 -> Scope/1, Sample and Hold/1  "q1*"
  S&H X3/2(y2) -> fbs/1, T DE PARK DIRECTA./2(fbs)
  S&H X3/1(y1) -> fas/1, T DE PARK DIRECTA./1(fas)
  S&H X3/3(y3) -> fcs/1, T DE PARK DIRECTA./3(fcs)
  Sample and Hold2/1 -> theta_m/1, Gain6/1  "y discreta"
  Pulse Generator2/1 -> Sample and Hold2/Trigger
  Pulse Generator1/1 -> Sample and Hold1/Trigger
  Sample and Hold1/1 -> MODULADOR DE TORQUE1/6(Ts)  "y discreta"
  Zero-Order Hold/1 -> Scope1/2, MODULAR DE TENSIÓN NO IDEAL/1(v_as*)  "con ZOH"
  Zero-Order Hold1/1 -> MODULAR DE TENSIÓN NO IDEAL/2(v_bs*)  "con ZOH"
  T DE PARK INVERSA/3(fcs) -> Zero-Order Hold2/1
  Zero-Order Hold2/1 -> MODULAR DE TENSIÓN NO IDEAL/3(v_cs*)  "con ZOH"
  T DE PARK INVERSA/2(fbs) -> Zero-Order Hold1/1
  T DE PARK INVERSA/1(fas) -> Scope1/1, Zero-Order Hold/1

== system Consigna5_2_1/Subsystem/Inversor: Modulador de tensión ==
  v_as* : Inport
  v_bs* : Inport  Port=2
  v_cs* : Inport  Port=3
  Gain5 : Gain
  Gain6 : Gain
  Gain7 : Gain
  v_as : Outport
  v_bs : Outport  Port=2
  v_cs : Outport  Port=3
  wires:
  v_as*/1 -> Gain5/1
  Gain5/1 -> v_as/1
  v_cs*/1 -> Gain7/1
  v_bs*/1 -> Gain6/1
  Gain7/1 -> v_cs/1
  Gain6/1 -> v_bs/1

== system Consigna5_2_1/Subsystem/Subsistema físico no lineal ==
  note: Retroalimentación natural del torque gravitacional
  T_per : Inport
  v_as : Inport  Port=2
  v_bs : Inport  Port=3
  v_cs : Inport  Port=4
  Tº_amb : Inport  Port=5
  Gain : Gain  Gain=P_p
  Gain1 : Gain  Gain=1/r
  Gain2 : Gain  Gain=k_l
  Gain3 : Gain  Gain=g
  Mux : Mux  Inputs=3
  Scope : Scope
  Sin : Trigonometry
  Subsistema electromagnético : Subsystem
      settings: PortSchema="{\"entries\":[{\"content\":{\"sides\":[{\"content\":{\"connectorIds\":[\"In1\",\"In2\",\"In3\",\"In4\"]},\"type\":\"ConnectorPlacement.EquallySpacedRectSide\",\"uuid\":\"c9fae60f-a644-4c7d-9a50-e330e891aba8\"},{\"content\":{\"connectorIds\":[\"Out1\",\"Out2\",\"Out3\",\"Out4\"],\"side\":\"RIGHT\"},\"type\":\"ConnectorPlacement.EquallySpacedRectSide\",\"uuid\":\"1bd25713-f5e9-4106-83eb-fb9f8a30d88e\"},{\"content\":{\"connectorIds\":[\"In5\"],\"side\":\"TOP\"},\"type\":\"ConnectorPlacement.EquallySpacedRectSide\",\"uuid\":\"c2f005dd-e04f-426d-b804-ce475aa5422d\"}]},\"type\":\"ConnectorPlacement.EquallySpacedConnector\",\"uuid\":\"9bdc4406-fcef-47cb-a5c0-d4f33f547a91\"}],\"packageUris\":[\"http://schema.mathworks.com/mf0/Connector/R2020b\"],\"version\":\"1.0\"}"
  Subsistema mecánico completo : Subsystem
  Subsistema térmico : Subsystem
  Sum : Sum  Inputs=++|
  TD_PARK : MATLAB Function  TreatAsAtomicUnit=on
  TI_PARK : MATLAB Function  TreatAsAtomicUnit=on
  theta_m : Outport
  T_s : Outport  Port=2
  i_abcs : Outport  Port=3
  r_s : Outport  Port=4
  T_m : Outport  Port=5
  omega_m : Outport  Port=6
  T_l : Outport  Port=7
  wires:
  Subsistema electromagnético/4(T_m) -> T_m/1, Subsistema mecánico completo/1(T_m)
  Subsistema electromagnético/3(i_0s) -> Subsistema térmico/3(i_0s^r), TI_PARK/3(f0s)
  Subsistema mecánico completo/2(omega_m(t)) -> Subsistema electromagnético/5(omega_m), Scope/1, omega_m/1
  Subsistema electromagnético/1(i_qs^r) -> Subsistema térmico/1(i_qs^r), TI_PARK/1(fqs)
  Subsistema electromagnético/2(i_ds^r) -> TI_PARK/2(fds), Subsistema térmico/2(i_ds^r)
  Sum/1 -> T_l/1, Subsistema mecánico completo/2(T_l)  "T_l"
  TD_PARK/1(fqs) -> Subsistema electromagnético/1(v_qs^r)
  Tº_amb/1 -> Subsistema térmico/4(Tº_amb)
  Mux/1 -> i_abcs/1
  TI_PARK/1(fas) -> Mux/1
  TI_PARK/2(fbs) -> Mux/2
  TI_PARK/3(fcs) -> Mux/3
  v_as/1 -> TD_PARK/1(fas)
  v_cs/1 -> TD_PARK/3(fcs)
  Gain/1 -> TI_PARK/4(theta_r), TD_PARK/4(theta_r)
  v_bs/1 -> TD_PARK/2(fbs)
  Gain1/1 -> Sin/1
  Sin/1 -> Gain2/1
  Gain2/1 -> Gain3/1
  T_per/1 -> Sum/2
  TD_PARK/2(fds) -> Subsistema electromagnético/2(v_ds^r)
  TD_PARK/3(f0s) -> Subsistema electromagnético/3(v_0s)
  Subsistema térmico/1(r_s) -> r_s/1, Subsistema electromagnético/4(r_s)
  Subsistema térmico/2(T_s) -> T_s/1
  Subsistema mecánico completo/1(theta_m(t)) -> theta_m/1, Gain1/1, Gain/1
  Gain3/1 -> Sum/1

== system Consigna5_2_1/Subsystem/Subsystem2 ==
  Tm* : Inport
  omega_m : Inport  Port=2
  R_s : Inport  Port=3
  i_qs^r : Inport  Port=4
  i_ds^r : Inport  Port=5
  i_0s : Inport  Port=6
  Constant5 : Constant  Value=0
  Desacoples Fisicos : Subsystem
  Lazo de Torque : Subsystem
  Modulador de corriente : Subsystem
  v_qs*' : Outport
  v_ds*' : Outport  Port=2
  v_0s*' : Outport  Port=3
  wires:
  Lazo de Torque/1(iqs*) -> Modulador de corriente/1(I_qs*)
  Modulador de corriente/3(v_0s*) -> Desacoples Fisicos/3(v_0s*)
  i_ds^r/1 -> Modulador de corriente/5(i_ds), Desacoples Fisicos/5(i_ds), Lazo de Torque/3(ids)
  Modulador de corriente/1(v_qs*) -> Desacoples Fisicos/1(v_qs*)
  Constant5/1 -> Modulador de corriente/2(I_ds*), Modulador de corriente/3(I_0s*)
  i_qs^r/1 -> Desacoples Fisicos/4(i_qs), Modulador de corriente/4(i_qs)
  Tm*/1 -> Lazo de Torque/1(Tm*)
  omega_m/1 -> Desacoples Fisicos/7(omega_m), Lazo de Torque/2(omega_m)
  Modulador de corriente/2(v_ds*) -> Desacoples Fisicos/2(v_ds*)
  i_0s/1 -> Desacoples Fisicos/6(i_0s), Modulador de corriente/6(i_0s)
  Desacoples Fisicos/2(v_ds*') -> v_ds*'/1
  Desacoples Fisicos/1(v_qs*') -> v_qs*'/1
  Desacoples Fisicos/3(v_0s*') -> v_0s*'/1
  R_s/1 -> Desacoples Fisicos/8(R_s)

== system Consigna5_2_1/Subsystem1/Controlador PID ==
  note: ba: Proporcional al error de velocidad
  note: Ksa: Proporcional a la integral al error de velocidad
  note: Ksia: Porporcional a la doble Integral al error de velocidad
  omega_m* : Inport
  omega_m : Inport  Port=2
  Gain : Gain  Gain=ba
  Gain1 : Gain  Gain=Ksa
  Gain2 : Gain  Gain=Ksia
  Integrator : Integrator
  Integrator1 : Integrator
  Sum : Sum  Inputs=|+-
  Sum1 : Sum  Inputs=+++
  Tm* : Outport
  wires:
  omega_m*/1 -> Sum/1
  omega_m/1 -> Sum/2
  Sum/1 -> Integrator/1, Gain/1
  Integrator/1 -> Integrator1/1, Gain1/1
  Gain/1 -> Sum1/3
  Sum1/1 -> Tm*/1
  Gain1/1 -> Sum1/2
  Integrator1/1 -> Gain2/1
  Gain2/1 -> Sum1/1

== system Consigna5_2_1/Subsystem1/Inversor: Modulador de tensión ==
  v_as* : Inport
  v_bs* : Inport  Port=2
  v_cs* : Inport  Port=3
  Gain5 : Gain
  Gain6 : Gain
  Gain7 : Gain
  v_as : Outport
  v_bs : Outport  Port=2
  v_cs : Outport  Port=3
  wires:
  v_as*/1 -> Gain5/1
  Gain5/1 -> v_as/1
  v_cs*/1 -> Gain7/1
  v_bs*/1 -> Gain6/1
  Gain7/1 -> v_cs/1
  Gain6/1 -> v_bs/1

== system Consigna5_2_1/Subsystem1/MODULADOR DE TORQUE1 ==
  Tm* : Inport
  omega_m : Inport  Port=2
  i_qs^r : Inport  Port=3
  i_ds^r : Inport  Port=4
  i_0s : Inport  Port=5
  Ts : Inport  Port=6
  Calculo rs : Subsystem
  Constant5 : Constant  Value=0
  Desacoples Fisicos : Subsystem
  Lazo de Torque : Subsystem
  Modulador de corriente : Subsystem
  v_qs*' : Outport
  v_ds*' : Outport  Port=2
  v_0s*' : Outport  Port=3
  wires:
  Lazo de Torque/1(iqs*) -> Modulador de corriente/1(I_qs*)
  Modulador de corriente/3(v_0s*) -> Desacoples Fisicos/3(v_0s*)
  i_ds^r/1 -> Modulador de corriente/5(i_ds), Desacoples Fisicos/5(i_ds), Lazo de Torque/3(ids)
  Modulador de corriente/1(v_qs*) -> Desacoples Fisicos/1(v_qs*)
  Constant5/1 -> Modulador de corriente/2(I_ds*), Modulador de corriente/3(I_0s*)
  i_qs^r/1 -> Desacoples Fisicos/4(i_qs), Modulador de corriente/4(i_qs)
  Tm*/1 -> Lazo de Torque/1(Tm*)
  omega_m/1 -> Desacoples Fisicos/7(omega_m), Lazo de Torque/2(omega_m)
  Modulador de corriente/2(v_ds*) -> Desacoples Fisicos/2(v_ds*)
  i_0s/1 -> Desacoples Fisicos/6(i_0s), Modulador de corriente/6(i_0s)
  Desacoples Fisicos/2(v_ds*') -> v_ds*'/1
  Desacoples Fisicos/1(v_qs*') -> v_qs*'/1
  Desacoples Fisicos/3(v_0s*') -> v_0s*'/1
  Ts/1 -> Calculo rs/1(Ts)
  Calculo rs/1(r_s) -> Desacoples Fisicos/8(R_s)
